simulink model "Example1Heart"  (R2025b)
settings: Solver=VariableStepAuto  StartTime=0.0  StopTime=10.0  RelTol=1e-3
libraries: Libs x7
settings Model: Creator=rfen801  LastModifiedBy=rfen801

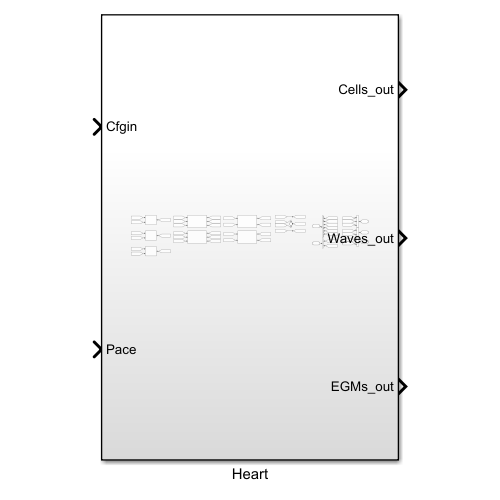
[thumbnail: Simulink's stored preview of the top-level diagram]
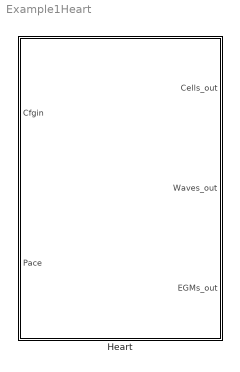
== system Example1Heart ==
  Heart : Subsystem

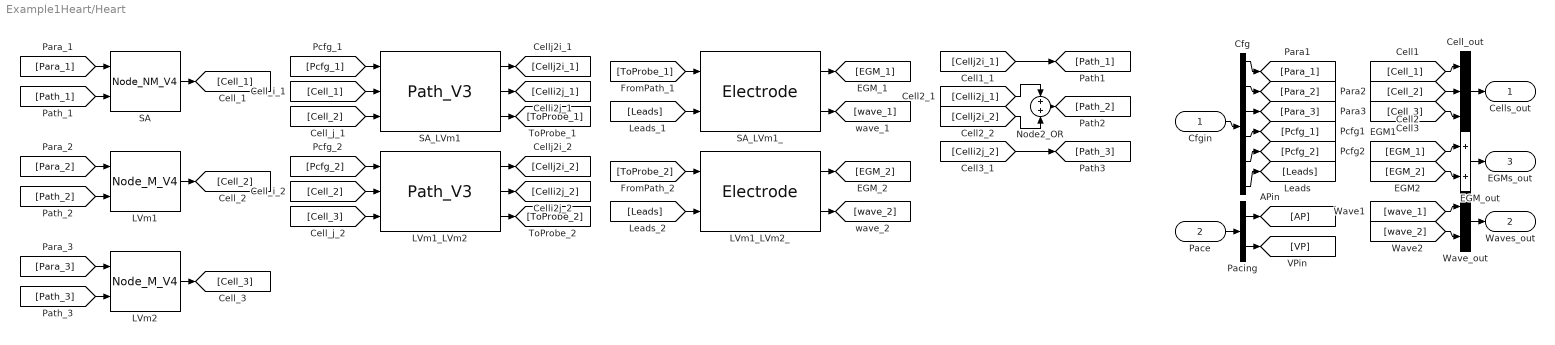
== system Example1Heart/Heart ==
  Cfgin : Inport
  Pace : Inport  Port=2
  Cell_out : Mux  Inputs=3
  Cfg : Demux  Outputs=[23,25,25,11,11,28]
  EGM_out : Sum  Inputs=2
  LVm1 : Libs/Node_M_V4  SystemSampleTime=-1  VariantActivationTime=update diagram  EmptyChoice=off  PassThrough=off  PassThroughVariantControl=(default)  EmptyChoiceVariantControl=(default)  AllowFlexibleInterface=on  Latency=0  AutoFrameSizeCalculation=off
  LVm1_LVm2 : Libs/Path_V3  SystemSampleTime=-1  VariantActivationTime=update diagram  EmptyChoice=off  PassThrough=off  PassThroughVariantControl=(default)  EmptyChoiceVariantControl=(default)  AllowFlexibleInterface=on  Latency=0  AutoFrameSizeCalculation=off
  LVm1_LVm2_ : Libs/Electrode  SystemSampleTime=-1  VariantActivationTime=update diagram  EmptyChoice=off  PassThrough=off  PassThroughVariantControl=(default)  EmptyChoiceVariantControl=(default)  AllowFlexibleInterface=on  Latency=0  AutoFrameSizeCalculation=off
  LVm2 : Libs/Node_M_V4  SystemSampleTime=-1  VariantActivationTime=update diagram  EmptyChoice=off  PassThrough=off  PassThroughVariantControl=(default)  EmptyChoiceVariantControl=(default)  AllowFlexibleInterface=on  Latency=0  AutoFrameSizeCalculation=off
  Node2_OR : Sum  Inputs=2
  Pacing : Demux  Outputs=2
  SA : Libs/Node_NM_V4  SystemSampleTime=-1  VariantActivationTime=update diagram  EmptyChoice=off  PassThrough=off  PassThroughVariantControl=(default)  EmptyChoiceVariantControl=(default)  AllowFlexibleInterface=on  Latency=0  AutoFrameSizeCalculation=off
  SA_LVm1 : Libs/Path_V3  SystemSampleTime=-1  VariantActivationTime=update diagram  EmptyChoice=off  PassThrough=off  PassThroughVariantControl=(default)  EmptyChoiceVariantControl=(default)  AllowFlexibleInterface=on  Latency=0  AutoFrameSizeCalculation=off
  SA_LVm1_ : Libs/Electrode  SystemSampleTime=-1  VariantActivationTime=update diagram  EmptyChoice=off  PassThrough=off  PassThroughVariantControl=(default)  EmptyChoiceVariantControl=(default)  AllowFlexibleInterface=on  Latency=0  AutoFrameSizeCalculation=off
  Wave_out : Mux  Inputs=2
  Cells_out : Outport
  Waves_out : Outport  Port=2
  EGMs_out : Outport  Port=3
  wires:
  SA/1 -> [Cell_1]
  [Para_1] -> SA/1
  [Path_1] -> SA/2
  LVm1/1 -> [Cell_2]
  [Para_2] -> LVm1/1
  [Path_2] -> LVm1/2
  LVm2/1 -> [Cell_3]
  [Para_3] -> LVm2/1
  [Path_3] -> LVm2/2
  SA_LVm1/1 -> [Cellj2i_1]
  SA_LVm1/2 -> [Celli2j_1]
  SA_LVm1/3 -> [ToProbe_1]
  [Pcfg_1] -> SA_LVm1/1
  [Cell_1] -> SA_LVm1/2
  [Cell_2] -> SA_LVm1/3
  LVm1_LVm2/1 -> [Cellj2i_2]
  LVm1_LVm2/2 -> [Celli2j_2]
  LVm1_LVm2/3 -> [ToProbe_2]
  [Pcfg_2] -> LVm1_LVm2/1
  [Cell_2] -> LVm1_LVm2/2
  [Cell_3] -> LVm1_LVm2/3
  SA_LVm1_/1 -> [EGM_1]
  SA_LVm1_/2 -> [wave_1]
  [ToProbe_1] -> SA_LVm1_/1
  [Leads] -> SA_LVm1_/2
  LVm1_LVm2_/1 -> [EGM_2]
  LVm1_LVm2_/2 -> [wave_2]
  [ToProbe_2] -> LVm1_LVm2_/1
  [Leads] -> LVm1_LVm2_/2
  [Cellj2i_1] -> [Path_1]
  [Celli2j_1] -> Node2_OR/1
  [Cellj2i_2] -> Node2_OR/2
  Node2_OR/1 -> [Path_2]
  [Celli2j_2] -> [Path_3]
  Cfgin/1 -> Cfg/1
  Pace/1 -> Pacing/1
  Cfg/1 -> [Para_1]
  Cfg/2 -> [Para_2]
  Cfg/3 -> [Para_3]
  Cfg/4 -> [Pcfg_1]
  Cfg/5 -> [Pcfg_2]
  Cfg/6 -> [Leads]
  Pacing/1 -> [AP]
  Pacing/2 -> [VP]
  Cell_out/1 -> Cells_out/1
  EGM_out/1 -> EGMs_out/1
  Wave_out/1 -> Waves_out/1
  [Cell_1] -> Cell_out/1
  [Cell_2] -> Cell_out/2
  [Cell_3] -> Cell_out/3
  [EGM_1] -> EGM_out/1
  [EGM_2] -> EGM_out/2
  [wave_1] -> Wave_out/1
  [wave_2] -> Wave_out/2
